simulink library "downlink_4c2t_foldingcfr_3firs_lib"  (Simulink 8.7)
settings: Solver=ode45  StartTime=0.0  StopTime=10.0  RelTol=1e-3
undefined symbols (not defined in the file or in its folder): AdvDSPBChannelOutDisplay, Anti, cfr_Params, dpoly, dspba_ChannelInVis, dspba_ChannelOutVis, dspba_internal_get_channel_ports, evalAionMaskParam, Folding, latency, primtype, REG, Symmetrical, value
undefined symbols (not defined in the file): cfr0_id, cfr_angle_cord_bits, cfr_angle_cord_fractional_bits, cfr_stages, cfr_xy_cord_bits, cfr_xy_cord_fractional_bits, clock_rate, DUC_LINEUP_param, REG_dut_id_addr, sample_rate
libraries: DSPBAPrim x74, CORDIC_lib x18, FoldingCFR_3FIRs_lib x16, DSPBAFilters x4, DSPBAModelBus x3, DSPBABase x3
(part 1 of 2)
settings Model: Creator=nsafari  LastModifiedBy=5g

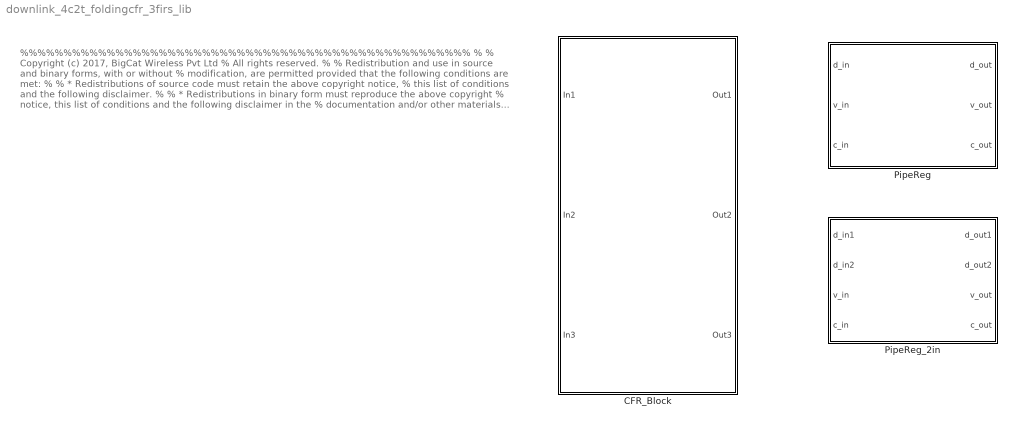
== system downlink_4c2t_foldingcfr_3firs_lib ==
  note: %%%%%%%%%%%%%%%%%%%%%%%%%%%%%%%%%%%%%%%%%%%%%%%%%%%%
      |  %
      |  % Copyright (c) 2017, BigCat Wireless Pvt Ltd
      |  % All rights reserved.
      |  %
      |  % Redistribution and use in source and binary forms, with or without
      |  % modification, are permitted provided that the following conditions are met:
      |  %
      |  %     * Redistributions of source code must retain the above copyright notice,
      |  %       this list of conditions and the following disclaimer.
      |  %
      |  %     * Redistributions in binary form must reproduce the above copyright
      |  %       notice, this list of conditions and the following disclaimer in the
      |  %       documentation and/or other materials provided with the distribution.
      |  %
      |  %     * Neither the name of the copyright holder nor the names of its contributors
      |  %       may be used to endorse or promote products derived from this software
      |  %       without specific prior written permission.
      |  %
      |  %
      |  %
      |  % THIS SOFTWARE IS PROVIDED BY THE COPYRIGHT HOLDERS AND CONTRIBUTORS "AS IS"
      |  % AND ANY EXPRESS OR IMPLIED WARRANTIES, INCLUDING, BUT NOT LIMITED TO, THE
      |  % IMPLIED WARRANTIES OF MERCHANTABILITY AND FITNESS FOR A PARTICULAR PURPOSE ARE
      |  % DISCLAIMED. IN NO EVENT SHALL THE COPYRIGHT HOLDER OR CONTRIBUTORS BE LIABLE
      |  % FOR ANY DIRECT, INDIRECT, INCIDENTAL, SPECIAL, EXEMPLARY, OR CONSEQUENTIAL
      |  % DAMAGES (INCLUDING, BUT NOT LIMITED TO, PROCUREMENT OF SUBSTITUTE GOODS OR
      |  % SERVICES; LOSS OF USE, DATA, OR PROFITS; OR BUSINESS INTERRUPTION) HOWEVER
      |  % CAUSED AND ON ANY THEORY OF LIABILITY, WHETHER IN CONTRACT, STRICT LIABILITY,
      |  % OR TORT (INCLUDING NEGLIGENCE OR OTHERWISE) ARISING IN ANY WAY OUT OF THE USE
      |  % OF THIS SOFTWARE, EVEN IF ADVISED OF THE POSSIBILITY OF SUCH DAMAGE.
      |  %
      |   %%%%%%%%%%%%%%%%%%%%%%%%%%%%%%%%%%%%%%%%%%%%%%%%%%%%%
  CFR_Block : Subsystem  AncestorBlock=CFR_library/CFR_Block  mask(Altera CFR Library Block){clk=clock_rate, sample_rate=sample_rate, Folding=Folding, block_id=cfr0_id, block_id_addr=REG_dut_id_addr, cfr_Params=cfr_Params, REG=REG}
      mask prompts: clk "System clock"; sample_rate "sample rate"; Folding "Folding Factor"; block_id "Unique ID of CFR"; block_id_addr "CFR ID address"; cfr_Params "CFR Configuration Structure"; REG "Register Map"
      mask help:
      | The block has the following parameters:
      |
      | "system clock" - the clock rate CFR module runs.
      |
      | "sample rate" - input signal sampling rate.
      |
      | "Folding Factor" - the number of folding for the module time-sharing;
      | It takes integer values between 1 and floor(system clock / sample rate).
      |
      | "Unique ID of CFR" is a unique numerical integer identifier for the CFR
      | block, this is used once the block is in a larger system to confirm the
      | correct block is being accessed.
      |
      | "CFR ID address" this is the relative address of the "Unique ID of CFR"
      | typically this is zero (at the CFR base address).
      |
      | "CFR Configuration Structure" - an array structure containing the
      | configuration of the CFR block. The length of this parameter specifies the
      | number of CFR core iterations instantiated.
      |
      | "Register Map" a structure containing the register map for CFR block.
      |
      | The settings of the above are exemplified in the setup script of the
      | altera_cfr example design.
      mask init:
      | %setup_cfr_block(iters, Iter_Params, REG, block_id, block_id_addr);
      mask Display:
      | color('w');
      | image(imread('dspba_prim.jpg'));
      | fprintf('FIR-based \n Peak Cancelling CFR \n \n Folding Factor: %d\n', Folding);
      | port_label('input',1,'valid');port_label('input',2,'channel');port_label('input',3,'xr');
      | port_label('output',1,'v');port_label('output',2,'c');port_label('output',3,'zr');
  PipeReg : Subsystem  mask{NPipe=2, Clock_Margin=DUC_LINEUP_param.ClockMargin}
      mask prompts: NPipe "Pipeline stages"; Clock_Margin "Clock Margin"
      mask Display:
      | d = strcat(num2str(NPipe), '\npipeline\nstages');
      | disp(d);
      | port_label('input',2,'v_in');
      | port_label('input',3,'c_in');
      | port_label('input',1,'d_in');
      | port_label('output',2,'v_out');
      | port_label('output',3,'c_out');
      | port_label('output',1,'d_out');
  PipeReg_2in : Subsystem  mask{NPipe=2, Clock_Margin=DUC_LINEUP_param.ClockMargin}
      mask prompts: NPipe "Pipeline stages"; Clock_Margin "Clock Margin"
      mask Display:
      | d = strcat(num2str(NPipe), '\npipeline\nstages');
      | disp(d);
      | port_label('input',3,'v_in');
      | port_label('input',4,'c_in');
      | port_label('input',1,'d_in1');
      | port_label('input',2,'d_in2');
      | port_label('output',3,'v_out');
      | port_label('output',4,'c_out');
      | port_label('output',1,'d_out1');
      | port_label('output',2,'d_out2');

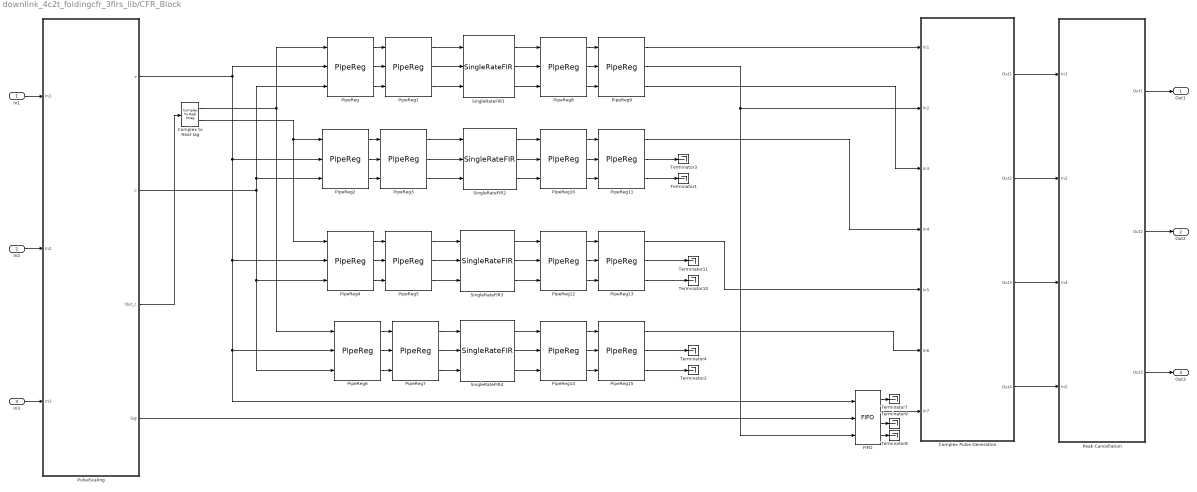
== system downlink_4c2t_foldingcfr_3firs_lib/CFR_Block ==
  In1 : Inport
  In2 : Inport  Port=2
  In3 : Inport  Port=3
  Complex Pulse Generation : Subsystem
  Complex to Real-Iag : ComplexToRealImag
  FIFO : DSPBAPrim/FIFO  primtype=fifo  nInputs=3  nOutputs=4  omode=Inherit via internal rule  otype=sfix(16)  scale=2^-15  rndmethod=Unbiased  factor=1  satmethod=Symmetric  shift_vec=[0 1 2 -1]  value=[16 8 16]  inPortNames=['w'; 'd'; 'r'; 'f']  outPortNames=['v'; 'q'; 't'; 'f']  dspbaimage=dspba_prim.jpg  text=fprintf('fifo');  style=Optimised  visibilities=263168  version=20130808  user_sclr=off
  Peak Cancellation : Subsystem
  PipeReg{,1..15} (16 alike) : FoldingCFR_3FIRs_lib/PipeReg  NPipe=2  Clock_Margin=DUC_LINEUP_param.ClockMargin
  PulseScaling : Subsystem
  SingleRateFIR1 : DSPBAFilters/SingleRateFIR  nInputRate=sample_rate  nchan=Folding  symmetry=Symmetrical  coef=fi(cfr_Params.firCOEF1,1,16,15)  addr=cfr_Params.BaseAddr + REG.FirTap1  rwmode=Read/Write  nband=Use All Taps  latency=3  exposebus=off  version=20090407
      settings: AttributesFormatString=%<latency>
  SingleRateFIR2 : DSPBAFilters/SingleRateFIR  nInputRate=sample_rate  nchan=Folding  symmetry=Anti-Symmetrical  coef=fi(cfr_Params.firCOEF2,1,16,15)  addr=cfr_Params.BaseAddr + REG.FirTap2  rwmode=Read/Write  nband=Use All Taps  latency=3  exposebus=off  version=20090407
  SingleRateFIR3 : DSPBAFilters/SingleRateFIR  nInputRate=sample_rate  nchan=Folding  symmetry=Symmetrical  coef=fi(cfr_Params.firCOEF3,1,16,15)  addr=cfr_Params.BaseAddr + REG.FirTap3  rwmode=Read/Write  nband=Use All Taps  latency=3  exposebus=off  version=20090407
  SingleRateFIR4 : DSPBAFilters/SingleRateFIR  nInputRate=sample_rate  nchan=Folding  symmetry=Anti-Symmetrical  coef=fi(cfr_Params.firCOEF4,1,16,15)  addr=cfr_Params.BaseAddr + REG.FirTap4  rwmode=Read/Write  nband=Use All Taps  latency=3  exposebus=off  version=20090407
  Terminator{1..4,7..11} (9 alike) : Terminator
  Out1 : Outport
  Out2 : Outport  Port=2
  Out3 : Outport  Port=3
  wires:
  In1/1 -> PulseScaling/1(In1)
  In2/1 -> PulseScaling/2(In2)
  In3/1 -> PulseScaling/3(In3)
  Peak Cancellation/1(Out1) -> Out1/1
  Peak Cancellation/2(Out2) -> Out2/1
  Peak Cancellation/3(Out3) -> Out3/1
  FIFO/1 -> Terminator7/1
  FIFO/4 -> Terminator8/1
  FIFO/3 -> Terminator9/1
  PulseScaling/3(Out_c) -> Complex to Real-Iag/1
  FIFO/2 -> Complex Pulse Generation/7(In7)
  Complex Pulse Generation/1(Out1) -> Peak Cancellation/1(In1)
  Complex Pulse Generation/3(Out3) -> Peak Cancellation/3(In4)
  Complex Pulse Generation/4(Out4) -> Peak Cancellation/4(In5)
  Complex Pulse Generation/2(Out2) -> Peak Cancellation/2(In2)
  Complex to Real-Iag/2 -> PipeReg4/1, PipeReg2/1
  Complex to Real-Iag/1 -> PipeReg6/1, PipeReg/1
  PulseScaling/2(c) -> PipeReg2/3, PipeReg/3, PipeReg6/3, PipeReg4/3
  PulseScaling/1(v) -> PipeReg/2, PipeReg4/2, PipeReg6/2, FIFO/1, PipeReg2/2
  PulseScaling/4(Sig) -> FIFO/2
  PipeReg9/3 -> Complex Pulse Generation/3(In3)
  PipeReg9/1 -> Complex Pulse Generation/1(In1)
  PipeReg9/2 -> FIFO/3, Complex Pulse Generation/2(In2)
  PipeReg11/1 -> Complex Pulse Generation/4(In4)
  PipeReg11/3 -> Terminator1/1
  PipeReg11/2 -> Terminator3/1
  PipeReg13/1 -> Complex Pulse Generation/5(In5)
  PipeReg13/3 -> Terminator10/1
  PipeReg13/2 -> Terminator11/1
  PipeReg15/1 -> Complex Pulse Generation/6(In6)
  PipeReg15/3 -> Terminator2/1
  PipeReg15/2 -> Terminator4/1
  PipeReg/3 -> PipeReg1/3
  PipeReg/1 -> PipeReg1/1
  PipeReg/2 -> PipeReg1/2
  PipeReg1/2 -> SingleRateFIR1/2
  PipeReg1/1 -> SingleRateFIR1/1
  PipeReg1/3 -> SingleRateFIR1/3
  PipeReg2/3 -> PipeReg3/3
  PipeReg2/1 -> PipeReg3/1
  PipeReg2/2 -> PipeReg3/2
  PipeReg3/1 -> SingleRateFIR2/1
  PipeReg3/2 -> SingleRateFIR2/2
  PipeReg3/3 -> SingleRateFIR2/3
  PipeReg4/3 -> PipeReg5/3
  PipeReg4/1 -> PipeReg5/1
  PipeReg4/2 -> PipeReg5/2
  PipeReg5/3 -> SingleRateFIR3/3
  PipeReg5/1 -> SingleRateFIR3/1
  PipeReg5/2 -> SingleRateFIR3/2
  PipeReg6/3 -> PipeReg7/3
  PipeReg6/1 -> PipeReg7/1
  PipeReg6/2 -> PipeReg7/2
  PipeReg7/1 -> SingleRateFIR4/1
  PipeReg7/2 -> SingleRateFIR4/2
  PipeReg7/3 -> SingleRateFIR4/3
  PipeReg8/3 -> PipeReg9/3
  PipeReg8/1 -> PipeReg9/1
  PipeReg8/2 -> PipeReg9/2
  SingleRateFIR1/1 -> PipeReg8/1
  SingleRateFIR1/3 -> PipeReg8/3
  SingleRateFIR1/2 -> PipeReg8/2
  PipeReg10/3 -> PipeReg11/3
  PipeReg10/1 -> PipeReg11/1
  PipeReg10/2 -> PipeReg11/2
  SingleRateFIR2/1 -> PipeReg10/1
  SingleRateFIR2/2 -> PipeReg10/2
  SingleRateFIR2/3 -> PipeReg10/3
  PipeReg12/3 -> PipeReg13/3
  PipeReg12/1 -> PipeReg13/1
  PipeReg12/2 -> PipeReg13/2
  SingleRateFIR3/2 -> PipeReg12/2
  SingleRateFIR3/1 -> PipeReg12/1
  SingleRateFIR3/3 -> PipeReg12/3
  PipeReg14/3 -> PipeReg15/3
  PipeReg14/1 -> PipeReg15/1
  PipeReg14/2 -> PipeReg15/2
  SingleRateFIR4/1 -> PipeReg14/1
  SingleRateFIR4/3 -> PipeReg14/3
  SingleRateFIR4/2 -> PipeReg14/2

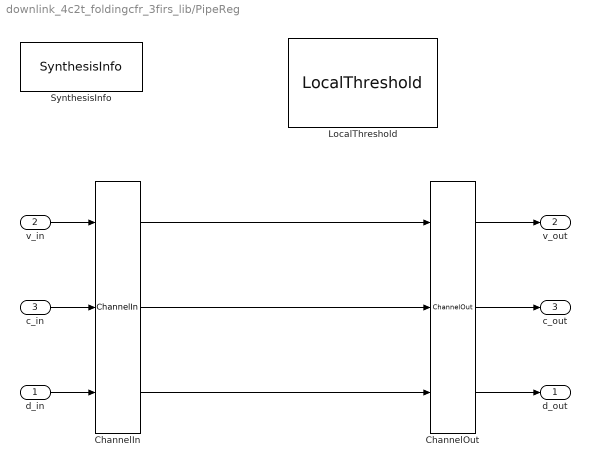
== system downlink_4c2t_foldingcfr_3firs_lib/PipeReg ==
  d_in : Inport
  v_in : Inport  Port=2
  c_in : Inport  Port=3
  ChannelIn : DSPBAPrim/ChannelIn  primtype=channelin  nInputs=dspba_internal_get_channel_ports(gcb)  nOutputs=dspba_internal_get_channel_ports(gcb)  omode=Inherit via internal rule  otype=sfix(16)  scale=2^-15  rndmethod=Unbiased  factor=1  satmethod=Symmetric  shift_vec=[0 1 2 -1]  value=1  inPortNames=['v'; 'c'; '0'; '1'; '2'; '3'; '4'; '5'; '6'; '7'; '8'; '9'; 'A'; 'B'; 'D'; 'E'; 'F'; 'G'; 'H'; 'I'; 'J'; 'K'; 'L'; 'M'; 'N'; 'O'; 'P'; 'Q'; 'R'; 'S'; 'T'; 'U'; 'W'; 'X'; 'Y'; 'Z']  outPortNames=['v'; 'c'; '0'; '1'; '2'; '3'; '4'; '5'; '6'; '7'; '8'; '9'; 'A'; 'B'; 'D'; 'E'; 'F'; 'G'; 'H'; 'I'; 'J'; 'K'; 'L'; 'M'; 'N'; 'O'; 'P'; 'Q'; 'R'; 'S'; 'T'; 'U'; 'W'; 'X'; 'Y'; 'Z']  dspbaimage=dspba_prim.jpg  text=fprintf('In');  style=Optimised  dataSignals=1  foldingEnabled=off  channels=1  sampleRate=200  packetBeginPresent=off  packetBeginEnabled=off  visibilities=dspba_ChannelInVis(gcb)  latencyCorrection=0  version=20141013
  ChannelOut : DSPBAPrim/ChannelOut  primtype=channelout  nInputs=dspba_internal_get_channel_ports(gcb)  nOutputs=dspba_internal_get_channel_ports(gcb)  omode=Inherit via internal rule  otype=sfix(16)  scale=2^-15  rndmethod=Unbiased  factor=1  satmethod=Symmetric  shift_vec=[0 1 2 -1]  value=1  inPortNames=['v'; 'c'; '0'; '1'; '2'; '3'; '4'; '5'; '6'; '7'; '8'; '9'; 'A'; 'B'; 'D'; 'E'; 'F'; 'G'; 'H'; 'I'; 'J'; 'K'; 'L'; 'M'; 'N'; 'O'; 'P'; 'Q'; 'R'; 'S'; 'T'; 'U'; 'W'; 'X'; 'Y'; 'Z']  outPortNames=['v'; 'c'; '0'; '1'; '2'; '3'; '4'; '5'; '6'; '7'; '8'; '9'; 'A'; 'B'; 'D'; 'E'; 'F'; 'G'; 'H'; 'I'; 'J'; 'K'; 'L'; 'M'; 'N'; 'O'; 'P'; 'Q'; 'R'; 'S'; 'T'; 'U'; 'W'; 'X'; 'Y'; 'Z']  dspbaimage=dspba_prim.jpg  text=fprintf('Out%s', AdvDSPBChannelOutDisplay(latency));  style=Optimised  dataSignals=1  foldingEnabled=off  channels=1  sampleRate=200  packetBeginPresent=off  packetBeginEnabled=off  visibilities=dspba_ChannelOutVis(gcb)  latency=2  latencyCorrection=0  version=20141013
  LocalThreshold : DSPBABase/LocalThreshold  margin=Clock_Margin  delayRegOrRAMThresholdBits=10000  MediumDualMemThresholdBits=-1  LargeDualMemThresholdBits=-1  hardMultiplierThresholdLuts=-1  version=0
  SynthesisInfo : DSPBAPrim/SynthesisInfo  primtype=synthinfo  nInputs=0  nOutputs=0  omode=Inherit via internal rule  otype=sfix(16)  scale=2^-15  rndmethod=Truncate  factor=1  satmethod=Symmetric  shift_vec=[0 1 2 -1]  value=99  inPortNames=[' '; ' ';]  outPortNames=[' ']  dspbaimage=dspba_prim.jpg  text=fprintf('Style=%s', style);  style=Scheduled  visibilities=32768  constraintInUse=on  constraintRelation==  constraintLimit=NPipe  bitAccurate=off  version=20090407
  d_out : Outport
  v_out : Outport  Port=2
  c_out : Outport  Port=3
  wires:
  ChannelOut/2 -> c_out/1
  ChannelOut/1 -> v_out/1
  ChannelOut/3 -> d_out/1
  c_in/1 -> ChannelIn/2
  v_in/1 -> ChannelIn/1
  ChannelIn/2 -> ChannelOut/2
  d_in/1 -> ChannelIn/3
  ChannelIn/1 -> ChannelOut/1
  ChannelIn/3 -> ChannelOut/3

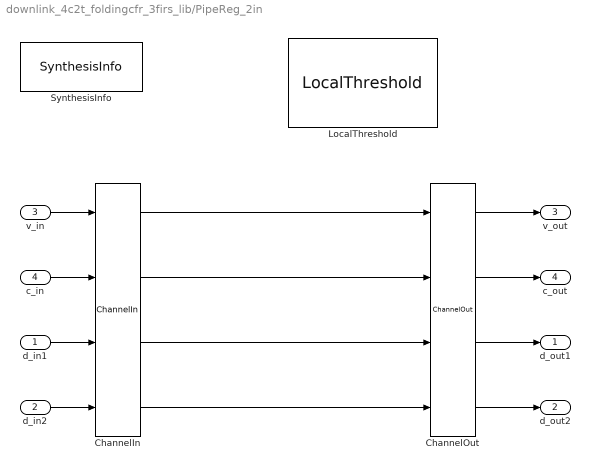
== system downlink_4c2t_foldingcfr_3firs_lib/PipeReg_2in ==
  d_in1 : Inport
  d_in2 : Inport  Port=2
  v_in : Inport  Port=3
  c_in : Inport  Port=4
  ChannelIn : DSPBAPrim/ChannelIn  primtype=channelin  nInputs=dspba_internal_get_channel_ports(gcb)  nOutputs=dspba_internal_get_channel_ports(gcb)  omode=Inherit via internal rule  otype=sfix(16)  scale=2^-15  rndmethod=Unbiased  factor=1  satmethod=Symmetric  shift_vec=[0 1 2 -1]  value=2  inPortNames=['v'; 'c'; '0'; '1'; '2'; '3'; '4'; '5'; '6'; '7'; '8'; '9'; 'A'; 'B'; 'D'; 'E'; 'F'; 'G'; 'H'; 'I'; 'J'; 'K'; 'L'; 'M'; 'N'; 'O'; 'P'; 'Q'; 'R'; 'S'; 'T'; 'U'; 'W'; 'X'; 'Y'; 'Z']  outPortNames=['v'; 'c'; '0'; '1'; '2'; '3'; '4'; '5'; '6'; '7'; '8'; '9'; 'A'; 'B'; 'D'; 'E'; 'F'; 'G'; 'H'; 'I'; 'J'; 'K'; 'L'; 'M'; 'N'; 'O'; 'P'; 'Q'; 'R'; 'S'; 'T'; 'U'; 'W'; 'X'; 'Y'; 'Z']  dspbaimage=dspba_prim.jpg  text=fprintf('In');  style=Optimised  dataSignals=2  foldingEnabled=off  channels=1  sampleRate=200  packetBeginPresent=off  packetBeginEnabled=off  visibilities=dspba_ChannelInVis(gcb)  latencyCorrection=0  version=20141013
  ChannelOut : DSPBAPrim/ChannelOut  primtype=channelout  nInputs=dspba_internal_get_channel_ports(gcb)  nOutputs=dspba_internal_get_channel_ports(gcb)  omode=Inherit via internal rule  otype=sfix(16)  scale=2^-15  rndmethod=Unbiased  factor=1  satmethod=Symmetric  shift_vec=[0 1 2 -1]  value=2  inPortNames=['v'; 'c'; '0'; '1'; '2'; '3'; '4'; '5'; '6'; '7'; '8'; '9'; 'A'; 'B'; 'D'; 'E'; 'F'; 'G'; 'H'; 'I'; 'J'; 'K'; 'L'; 'M'; 'N'; 'O'; 'P'; 'Q'; 'R'; 'S'; 'T'; 'U'; 'W'; 'X'; 'Y'; 'Z']  outPortNames=['v'; 'c'; '0'; '1'; '2'; '3'; '4'; '5'; '6'; '7'; '8'; '9'; 'A'; 'B'; 'D'; 'E'; 'F'; 'G'; 'H'; 'I'; 'J'; 'K'; 'L'; 'M'; 'N'; 'O'; 'P'; 'Q'; 'R'; 'S'; 'T'; 'U'; 'W'; 'X'; 'Y'; 'Z']  dspbaimage=dspba_prim.jpg  text=fprintf('Out%s', AdvDSPBChannelOutDisplay(latency));  style=Optimised  dataSignals=2  foldingEnabled=off  channels=1  sampleRate=200  packetBeginPresent=off  packetBeginEnabled=off  visibilities=dspba_ChannelOutVis(gcb)  latency=2  latencyCorrection=0  version=20141013
  LocalThreshold : DSPBABase/LocalThreshold  margin=Clock_Margin  delayRegOrRAMThresholdBits=10000  MediumDualMemThresholdBits=-1  LargeDualMemThresholdBits=-1  hardMultiplierThresholdLuts=-1  version=0
  SynthesisInfo : DSPBAPrim/SynthesisInfo  primtype=synthinfo  nInputs=0  nOutputs=0  omode=Inherit via internal rule  otype=sfix(16)  scale=2^-15  rndmethod=Truncate  factor=1  satmethod=Symmetric  shift_vec=[0 1 2 -1]  value=99  inPortNames=[' '; ' ';]  outPortNames=[' ']  dspbaimage=dspba_prim.jpg  text=fprintf('Style=%s', style);  style=Scheduled  visibilities=32768  constraintInUse=on  constraintRelation==  constraintLimit=NPipe  bitAccurate=off  version=20090407
  "d_out1 " : Outport
  d_out2 : Outport  Port=2
  v_out : Outport  Port=3
  c_out : Outport  Port=4
  wires:
  ChannelIn/3 -> ChannelOut/3
  ChannelIn/1 -> ChannelOut/1
  d_in1/1 -> ChannelIn/3
  ChannelIn/2 -> ChannelOut/2
  v_in/1 -> ChannelIn/1
  c_in/1 -> ChannelIn/2
  ChannelOut/3 -> "d_out1 "/1
  ChannelOut/1 -> v_out/1
  ChannelOut/2 -> c_out/1
  d_in2/1 -> ChannelIn/4
  ChannelIn/4 -> ChannelOut/4
  ChannelOut/4 -> d_out2/1

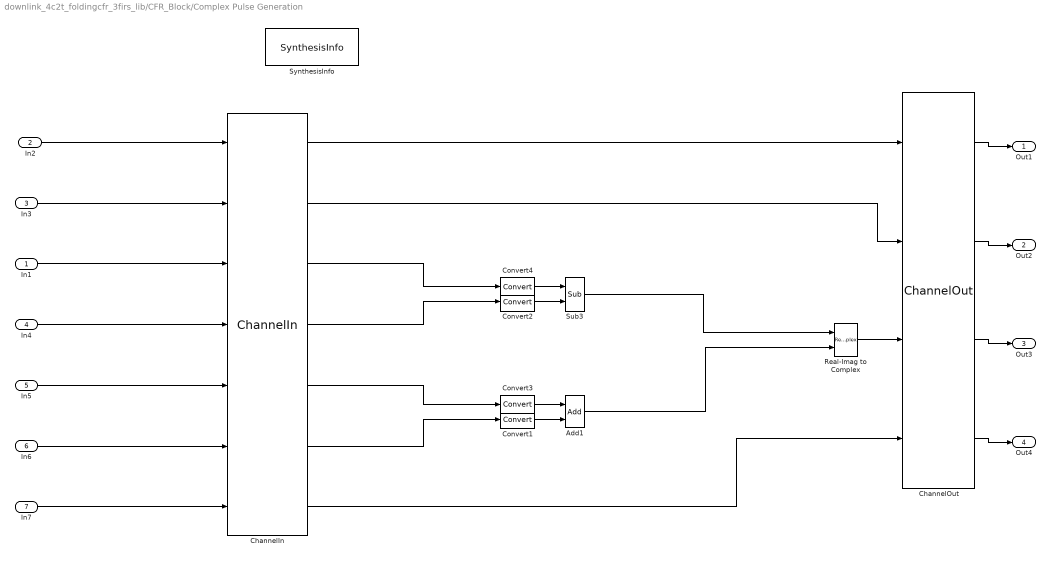
== system downlink_4c2t_foldingcfr_3firs_lib/CFR_Block/Complex Pulse Generation ==
  In1 : Inport
  In2 : Inport  Port=2
  In3 : Inport  Port=3
  In4 : Inport  Port=4
  In5 : Inport  Port=5
  In6 : Inport  Port=6
  In7 : Inport  Port=7
  Add1 : DSPBAPrim/Add  primtype=add  nInputs=evalAionMaskParam(gcb,'value',1)  nOutputs=1  omode=Inherit via internal rule with word growth  otype=sfix(16)  scale=2^-15  rndmethod=Unbiased  factor=1  satmethod=Symmetric  shift_vec=[0 1 2 -1]  value=2  inPortNames=[' '; ' ';]  outPortNames=[' ']  dspbaimage=dspba_prim.jpg  text=fprintf('+');  style=Optimised  visibilities=1032+2^17+2^18+2^19  genFPC=off  floatRounding=correct  advOptions=[]  version=20130821
  ChannelIn : DSPBAPrim/ChannelIn  primtype=channelin  nInputs=dspba_internal_get_channel_ports(gcb)  nOutputs=dspba_internal_get_channel_ports(gcb)  omode=Inherit via internal rule  otype=sfix(16)  scale=2^-15  rndmethod=Unbiased  factor=1  satmethod=Symmetric  shift_vec=[0 1 2 -1]  value=5  inPortNames=['v'; 'c'; '0'; '1'; '2'; '3'; '4'; '5'; '6'; '7'; '8'; '9'; 'A'; 'B'; 'D'; 'E'; 'F'; 'G'; 'H'; 'I'; 'J'; 'K'; 'L'; 'M'; 'N'; 'O'; 'P'; 'Q'; 'R'; 'S'; 'T'; 'U'; 'W'; 'X'; 'Y'; 'Z']  outPortNames=['v'; 'c'; '0'; '1'; '2'; '3'; '4'; '5'; '6'; '7'; '8'; '9'; 'A'; 'B'; 'D'; 'E'; 'F'; 'G'; 'H'; 'I'; 'J'; 'K'; 'L'; 'M'; 'N'; 'O'; 'P'; 'Q'; 'R'; 'S'; 'T'; 'U'; 'W'; 'X'; 'Y'; 'Z']  dspbaimage=dspba_prim.jpg  text=fprintf('In');  style=Optimised  dataSignals=5  foldingEnabled=off  channels=1  sampleRate=200  packetBeginPresent=off  packetBeginEnabled=off  visibilities=dspba_ChannelInVis(gcb)  latencyCorrection=0  version=20141013
  ChannelOut : DSPBAPrim/ChannelOut  primtype=channelout  nInputs=dspba_internal_get_channel_ports(gcb)  nOutputs=dspba_internal_get_channel_ports(gcb)  omode=Inherit via internal rule  otype=sfix(16)  scale=2^-15  rndmethod=Unbiased  factor=1  satmethod=Symmetric  shift_vec=[0 1 2 -1]  value=2  inPortNames=['v'; 'c'; '0'; '1'; '2'; '3'; '4'; '5'; '6'; '7'; '8'; '9'; 'A'; 'B'; 'D'; 'E'; 'F'; 'G'; 'H'; 'I'; 'J'; 'K'; 'L'; 'M'; 'N'; 'O'; 'P'; 'Q'; 'R'; 'S'; 'T'; 'U'; 'W'; 'X'; 'Y'; 'Z']  outPortNames=['v'; 'c'; '0'; '1'; '2'; '3'; '4'; '5'; '6'; '7'; '8'; '9'; 'A'; 'B'; 'D'; 'E'; 'F'; 'G'; 'H'; 'I'; 'J'; 'K'; 'L'; 'M'; 'N'; 'O'; 'P'; 'Q'; 'R'; 'S'; 'T'; 'U'; 'W'; 'X'; 'Y'; 'Z']  dspbaimage=dspba_prim.jpg  text=fprintf('Out%s', AdvDSPBChannelOutDisplay(latency));  style=Optimised  dataSignals=2  foldingEnabled=off  channels=1  sampleRate=200  packetBeginPresent=off  packetBeginEnabled=off  visibilities=dspba_ChannelOutVis(gcb)  latency=6  latencyCorrection=0  version=20141013
  Convert{1..4} (4 alike) : DSPBAPrim/Convert  primtype=convert  nInputs=1  nOutputs=1  omode=Specify via dialog  otype=sfix(16)  scale=2^-15  rndmethod=Unbiased  factor=1  satmethod=None  shift_vec=[0 1 2 -1]  value=round([0:255]/17)  inPortNames=[' '; ' ';]  outPortNames=[' '; 'c']  dspbaimage=dspba_prim.jpg  text=fprintf('convert');  style=Optimised  visibilities=8+64+256+2^17  clipdetect=off  floatPrecision=float32_m23  advOptions=[]  version=20130211
  Real-Imag to Complex : RealImagToComplex
  Sub3 : DSPBAPrim/Sub  primtype=sub  nInputs=2  nOutputs=1  omode=Inherit via internal rule with word growth  otype=sfix(16)  scale=2^-15  rndmethod=Unbiased  factor=1  satmethod=Symmetric  shift_vec=[0 1 2 -1]  value=0  inPortNames=['+'; '-';]  outPortNames=[' ']  dspbaimage=dspba_prim.jpg  text=fprintf('-');  style=Optimised  visibilities=8  floatRounding=correct  advOptions=[]  version=20130115
  SynthesisInfo : DSPBAPrim/SynthesisInfo  primtype=synthinfo  nInputs=0  nOutputs=0  omode=Inherit via internal rule  otype=sfix(16)  scale=2^-15  rndmethod=Truncate  factor=1  satmethod=Symmetric  shift_vec=[0 1 2 -1]  value=99  inPortNames=[' '; ' ';]  outPortNames=[' ']  dspbaimage=dspba_prim.jpg  text=fprintf('Style=%s', style);  style=Scheduled  visibilities=32768  constraintInUse=on  constraintRelation=>  constraintLimit=20  bitAccurate=off  version=20090407
  Out1 : Outport
  Out2 : Outport  Port=2
  Out3 : Outport  Port=3
  Out4 : Outport  Port=4
  wires:
  In1/1 -> ChannelIn/3
  ChannelIn/4 -> Convert2/1
  In4/1 -> ChannelIn/4
  ChannelIn/3 -> Convert4/1
  ChannelIn/6 -> Convert1/1
  In3/1 -> ChannelIn/2
  ChannelIn/1 -> ChannelOut/1
  ChannelIn/2 -> ChannelOut/2
  In7/1 -> ChannelIn/7
  ChannelIn/5 -> Convert3/1
  In5/1 -> ChannelIn/5
  In6/1 -> ChannelIn/6
  In2/1 -> ChannelIn/1
  ChannelIn/7 -> ChannelOut/4
  Sub3/1 -> Real-Imag to Complex/1
  ChannelOut/1 -> Out1/1
  ChannelOut/4 -> Out4/1
  ChannelOut/3 -> Out3/1
  Real-Imag to Complex/1 -> ChannelOut/3
  Add1/1 -> Real-Imag to Complex/2
  Convert1/1 -> Add1/2
  Convert3/1 -> Add1/1
  Convert2/1 -> Sub3/2
  Convert4/1 -> Sub3/1
  ChannelOut/2 -> Out2/1

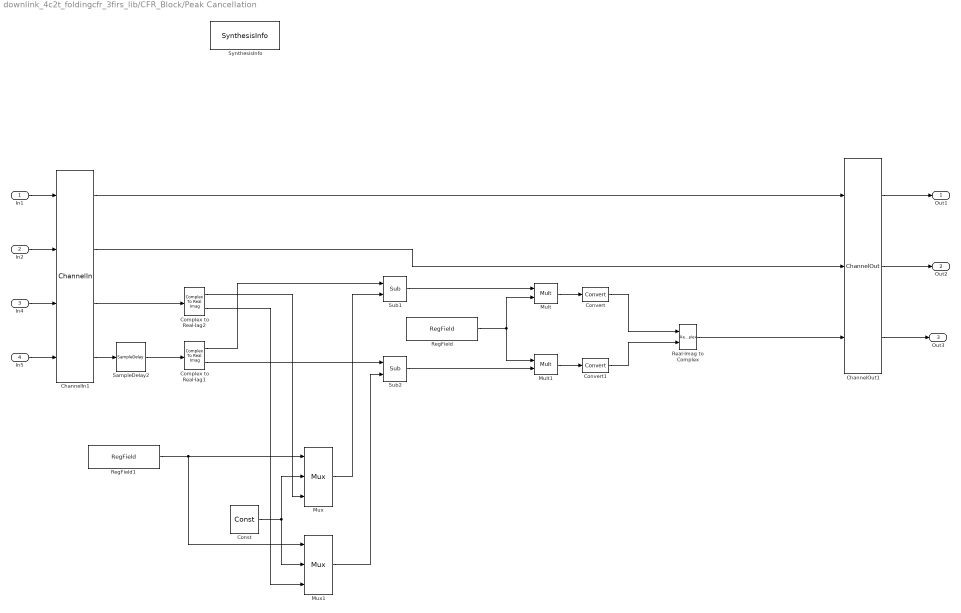
== system downlink_4c2t_foldingcfr_3firs_lib/CFR_Block/Peak Cancellation ==
  In1 : Inport
  In2 : Inport  Port=2
  In4 : Inport  Port=3
  In5 : Inport  Port=4
  ChannelIn1 : DSPBAPrim/ChannelIn  primtype=channelin  nInputs=dspba_internal_get_channel_ports(gcb)  nOutputs=dspba_internal_get_channel_ports(gcb)  omode=Inherit via internal rule  otype=sfix(16)  scale=2^-15  rndmethod=Unbiased  factor=1  satmethod=Symmetric  shift_vec=[0 1 2 -1]  value=2  inPortNames=['v'; 'c'; '0'; '1'; '2'; '3'; '4'; '5'; '6'; '7'; '8'; '9'; 'A'; 'B'; 'D'; 'E'; 'F'; 'G'; 'H'; 'I'; 'J'; 'K'; 'L'; 'M'; 'N'; 'O'; 'P'; 'Q'; 'R'; 'S'; 'T'; 'U'; 'W'; 'X'; 'Y'; 'Z']  outPortNames=['v'; 'c'; '0'; '1'; '2'; '3'; '4'; '5'; '6'; '7'; '8'; '9'; 'A'; 'B'; 'D'; 'E'; 'F'; 'G'; 'H'; 'I'; 'J'; 'K'; 'L'; 'M'; 'N'; 'O'; 'P'; 'Q'; 'R'; 'S'; 'T'; 'U'; 'W'; 'X'; 'Y'; 'Z']  dspbaimage=dspba_prim.jpg  text=fprintf('In');  style=Optimised  dataSignals=2  foldingEnabled=off  channels=1  sampleRate=200  packetBeginPresent=off  packetBeginEnabled=off  visibilities=dspba_ChannelInVis(gcb)  latencyCorrection=0  version=20141013
  ChannelOut1 : DSPBAPrim/ChannelOut  primtype=channelout  nInputs=dspba_internal_get_channel_ports(gcb)  nOutputs=dspba_internal_get_channel_ports(gcb)  omode=Inherit via internal rule  otype=sfix(16)  scale=2^-15  rndmethod=Unbiased  factor=1  satmethod=Symmetric  shift_vec=[0 1 2 -1]  value=1  inPortNames=['v'; 'c'; '0'; '1'; '2'; '3'; '4'; '5'; '6'; '7'; '8'; '9'; 'A'; 'B'; 'D'; 'E'; 'F'; 'G'; 'H'; 'I'; 'J'; 'K'; 'L'; 'M'; 'N'; 'O'; 'P'; 'Q'; 'R'; 'S'; 'T'; 'U'; 'W'; 'X'; 'Y'; 'Z']  outPortNames=['v'; 'c'; '0'; '1'; '2'; '3'; '4'; '5'; '6'; '7'; '8'; '9'; 'A'; 'B'; 'D'; 'E'; 'F'; 'G'; 'H'; 'I'; 'J'; 'K'; 'L'; 'M'; 'N'; 'O'; 'P'; 'Q'; 'R'; 'S'; 'T'; 'U'; 'W'; 'X'; 'Y'; 'Z']  dspbaimage=dspba_prim.jpg  text=fprintf('Out%s', AdvDSPBChannelOutDisplay(latency));  style=Optimised  dataSignals=1  foldingEnabled=off  channels=1  sampleRate=200  packetBeginPresent=off  packetBeginEnabled=off  visibilities=dspba_ChannelOutVis(gcb)  latency=12  latencyCorrection=0  version=20141013
  Complex to Real-Iag1 : ComplexToRealImag
  Complex to Real-Iag2 : ComplexToRealImag
  Const : DSPBAPrim/Const  primtype=const  nInputs=0  nOutputs=1  omode=Inherit via internal rule  otype=sfix(16)  scale=2^-15  rndmethod=Unbiased  factor=1  satmethod=Symmetric  shift_vec=[0 1 2 -1]  value=0  inPortNames=['+'; '+';]  outPortNames=[' ']  dspbaimage=dspba_prim.jpg  text=fprintf('%s', num2str(value));  style=Optimised  visibilities=8 + 1024  floatPrecision=float32_m23  version=20120820
  Convert : DSPBAPrim/Convert  primtype=convert  nInputs=1  nOutputs=1  omode=Specify via dialog  otype=sfix(16)  scale=2^-15  rndmethod=Unbiased  factor=1  satmethod=None  shift_vec=[0 1 2 -1]  value=round([0:255]/17)  inPortNames=[' '; ' ';]  outPortNames=[' '; 'c']  dspbaimage=dspba_prim.jpg  text=fprintf('convert');  style=Optimised  visibilities=8+64+256+2^17  clipdetect=off  floatPrecision=float32_m23  advOptions=[]  version=20130211
  Convert1 : DSPBAPrim/Convert  primtype=convert  nInputs=1  nOutputs=1  omode=Specify via dialog  otype=sfix(16)  scale=2^-15  rndmethod=Unbiased  factor=1  satmethod=None  shift_vec=[0 1 2 -1]  value=round([0:255]/17)  inPortNames=[' '; ' ';]  outPortNames=[' '; 'c']  dspbaimage=dspba_prim.jpg  text=fprintf('convert');  style=Optimised  visibilities=8+64+256+2^17  clipdetect=off  floatPrecision=float32_m23  advOptions=[]  version=20130211
  Mult : DSPBAPrim/Mult  primtype=mult  nInputs=2  nOutputs=1  omode=Inherit via internal rule  otype=sfix(16)  scale=2^-15  rndmethod=Unbiased  factor=1  satmethod=Symmetric  shift_vec=[0 1 2 -1]  value=0  inPortNames=[' '; ' ';]  outPortNames=[' ']  dspbaimage=dspba_prim.jpg  text=fprintf('X');  style=Optimised  visibilities=8+2^18+2^19  floatPrecision=float32_m23  floatRounding=correct  advOptions=[]  version=20130115
  Mult1 : DSPBAPrim/Mult  primtype=mult  nInputs=2  nOutputs=1  omode=Inherit via internal rule  otype=sfix(16)  scale=2^-15  rndmethod=Unbiased  factor=1  satmethod=Symmetric  shift_vec=[0 1 2 -1]  value=0  inPortNames=[' '; ' ';]  outPortNames=[' ']  dspbaimage=dspba_prim.jpg  text=fprintf('X');  style=Optimised  visibilities=8+2^18+2^19  floatPrecision=float32_m23  floatRounding=correct  advOptions=[]  version=20130115
  Mux : DSPBAPrim/Mux  primtype=mux  nInputs=evalAionMaskParam(gcb,'value',1)+1  nOutputs=1  omode=Inherit via internal rule  otype=sfix(16)  scale=2^-15  rndmethod=Unbiased  factor=1  satmethod=Symmetric  shift_vec=[0 1 2 -1]  value=2  inPortNames=['s '; 'd0'; 'd1'; 'd2'; 'd3'; 'd4'; 'd5'; 'd6'; 'd7'; 'd8'; 'd9';]  outPortNames=[' ']  dspbaimage=dspba_prim.jpg  text=fprintf('%s', primtype);  style=Optimised  visibilities=1032  version=20131025
  Mux1 : DSPBAPrim/Mux  primtype=mux  nInputs=evalAionMaskParam(gcb,'value',1)+1  nOutputs=1  omode=Inherit via internal rule  otype=sfix(16)  scale=2^-15  rndmethod=Unbiased  factor=1  satmethod=Symmetric  shift_vec=[0 1 2 -1]  value=2  inPortNames=['s '; 'd0'; 'd1'; 'd2'; 'd3'; 'd4'; 'd5'; 'd6'; 'd7'; 'd8'; 'd9';]  outPortNames=[' ']  dspbaimage=dspba_prim.jpg  text=fprintf('%s', primtype);  style=Optimised  visibilities=1032  version=20131025
  Real-Imag to Complex : RealImagToComplex
  RegField : DSPBAModelBus/RegField  reg_name=cfr_Params.BaseAddr + REG.Scaling  reg_rwmode=Read/Write  reg_msb=15  reg_lsb=0  reg_mode=Specify via dialog  reg_type=ufix(16)  reg_scale=2^-12  reg_init=cfr_Params.Scaling  reg_desc=Scaling value  reg_modal=off  reg_desc0=0  reg_desc1=0  reg_desc2=0  reg_desc3=0  reg_desc4=0  reg_desc5=0  reg_desc6=0  reg_desc7=0  SampleTime=1  version=20090407
  RegField1 : DSPBAModelBus/RegField  reg_name=cfr_Params.BaseAddr + REG.Enable  reg_rwmode=Read/Write  reg_msb=0  reg_lsb=0  reg_mode=Specify via dialog  reg_type=ufix(1)  reg_scale=2^0  reg_init=cfr_Params.Enable  reg_desc=Enable CFR  reg_modal=off  reg_desc0=0  reg_desc1=0  reg_desc2=0  reg_desc3=0  reg_desc4=0  reg_desc5=0  reg_desc6=0  reg_desc7=0  SampleTime=1  version=20090407
  SampleDelay2 : DSPBAPrim/SampleDelay  primtype=sampdelay  nInputs=1  nOutputs=1  omode=Inherit via internal rule  otype=sfix(16)  scale=2^-15  rndmethod=Unbiased  factor=1  satmethod=Symmetric  shift_vec=[0 1 2 -1]  value=floor(length(cfr_Params.firCOEF1)/2)*Folding  inPortNames=[' '; ' ';]  outPortNames=[' ']  dspbaimage=dspba_prim.jpg  text=dpoly(1, eye(1,value+1), 'z')  style=Optimised  visibilities=8 + 1024 + 2^17 + 2^18  flexible=off  slackgroup=0  augmented=0  version=20090407  advOptions=[]
  Sub1 : DSPBAPrim/Sub  primtype=sub  nInputs=2  nOutputs=1  omode=Inherit via internal rule with word growth  otype=sfix(16)  scale=2^-15  rndmethod=Unbiased  factor=1  satmethod=Symmetric  shift_vec=[0 1 2 -1]  value=0  inPortNames=['+'; '-';]  outPortNames=[' ']  dspbaimage=dspba_prim.jpg  text=fprintf('-');  style=Optimised  visibilities=8  floatRounding=correct  advOptions=[]  version=20130115
  Sub2 : DSPBAPrim/Sub  primtype=sub  nInputs=2  nOutputs=1  omode=Inherit via internal rule with word growth  otype=sfix(16)  scale=2^-15  rndmethod=Unbiased  factor=1  satmethod=Symmetric  shift_vec=[0 1 2 -1]  value=0  inPortNames=['+'; '-';]  outPortNames=[' ']  dspbaimage=dspba_prim.jpg  text=fprintf('-');  style=Optimised  visibilities=8  floatRounding=correct  advOptions=[]  version=20130115
  SynthesisInfo : DSPBAPrim/SynthesisInfo  primtype=synthinfo  nInputs=0  nOutputs=0  omode=Inherit via internal rule  otype=sfix(16)  scale=2^-15  rndmethod=Truncate  factor=1  satmethod=Symmetric  shift_vec=[0 1 2 -1]  value=99  inPortNames=[' '; ' ';]  outPortNames=[' ']  dspbaimage=dspba_prim.jpg  text=fprintf('Style=%s', style);  style=Scheduled  visibilities=32768  constraintInUse=on  constraintRelation=>  constraintLimit=20  bitAccurate=off  version=20090407
  Out1 : Outport
  Out2 : Outport  Port=2
  Out3 : Outport  Port=3
  wires:
  ChannelIn1/3 -> Complex to Real-Iag2/1
  ChannelIn1/4 -> SampleDelay2/1
  Real-Imag to Complex/1 -> ChannelOut1/3
  ChannelIn1/1 -> ChannelOut1/1
  ChannelIn1/2 -> ChannelOut1/2
  In1/1 -> ChannelIn1/1
  In4/1 -> ChannelIn1/3
  In2/1 -> ChannelIn1/2
  In5/1 -> ChannelIn1/4
  ChannelOut1/1 -> Out1/1
  ChannelOut1/2 -> Out2/1
  ChannelOut1/3 -> Out3/1
  SampleDelay2/1 -> Complex to Real-Iag1/1
  RegField/1 -> Mult1/1, Mult/2
  Mult/1 -> Convert/1
  Mult1/1 -> Convert1/1
  Sub1/1 -> Mult/1
  Sub2/1 -> Mult1/2
  Convert/1 -> Real-Imag to Complex/1
  Convert1/1 -> Real-Imag to Complex/2
  RegField1/1 -> Mux/1, Mux1/1
  Complex to Real-Iag2/1 -> Mux/3
  Complex to Real-Iag2/2 -> Mux1/3
  Mux/1 -> Sub1/2
  Mux1/1 -> Sub2/2
  Const/1 -> Mux1/2, Mux/2
  Complex to Real-Iag1/1 -> Sub1/1
  Complex to Real-Iag1/2 -> Sub2/1

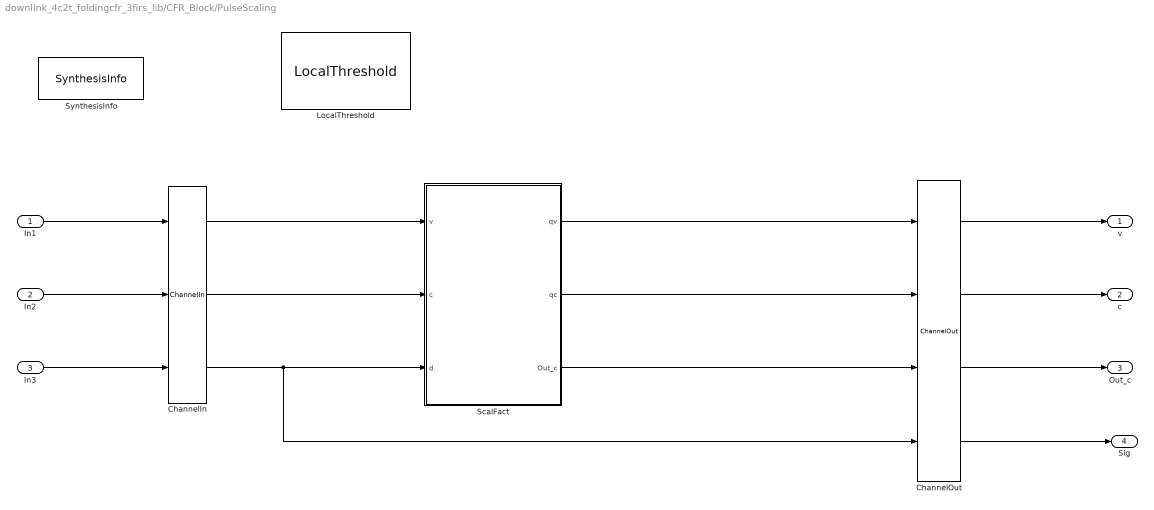
== system downlink_4c2t_foldingcfr_3firs_lib/CFR_Block/PulseScaling ==
  In1 : Inport
  In2 : Inport  Port=2
  In3 : Inport  Port=3
  ChannelIn : DSPBAPrim/ChannelIn  primtype=channelin  nInputs=dspba_internal_get_channel_ports(gcb)  nOutputs=dspba_internal_get_channel_ports(gcb)  omode=Inherit via internal rule  otype=sfix(16)  scale=2^-15  rndmethod=Unbiased  factor=1  satmethod=Symmetric  shift_vec=[0 1 2 -1]  value=1  inPortNames=['v'; 'c'; '0'; '1'; '2'; '3'; '4'; '5'; '6'; '7'; '8'; '9'; 'A'; 'B'; 'D'; 'E'; 'F'; 'G'; 'H'; 'I'; 'J'; 'K'; 'L'; 'M'; 'N'; 'O'; 'P'; 'Q'; 'R'; 'S'; 'T'; 'U'; 'W'; 'X'; 'Y'; 'Z']  outPortNames=['v'; 'c'; '0'; '1'; '2'; '3'; '4'; '5'; '6'; '7'; '8'; '9'; 'A'; 'B'; 'D'; 'E'; 'F'; 'G'; 'H'; 'I'; 'J'; 'K'; 'L'; 'M'; 'N'; 'O'; 'P'; 'Q'; 'R'; 'S'; 'T'; 'U'; 'W'; 'X'; 'Y'; 'Z']  dspbaimage=dspba_prim.jpg  text=fprintf('In');  style=Optimised  dataSignals=1  foldingEnabled=off  channels=1  sampleRate=200  packetBeginPresent=off  packetBeginEnabled=off  visibilities=dspba_ChannelInVis(gcb)  latencyCorrection=0  version=20141013
  ChannelOut : DSPBAPrim/ChannelOut  primtype=channelout  nInputs=dspba_internal_get_channel_ports(gcb)  nOutputs=dspba_internal_get_channel_ports(gcb)  omode=Inherit via internal rule  otype=sfix(16)  scale=2^-15  rndmethod=Unbiased  factor=1  satmethod=Symmetric  shift_vec=[0 1 2 -1]  value=2  inPortNames=['v'; 'c'; '0'; '1'; '2'; '3'; '4'; '5'; '6'; '7'; '8'; '9'; 'A'; 'B'; 'D'; 'E'; 'F'; 'G'; 'H'; 'I'; 'J'; 'K'; 'L'; 'M'; 'N'; 'O'; 'P'; 'Q'; 'R'; 'S'; 'T'; 'U'; 'W'; 'X'; 'Y'; 'Z']  outPortNames=['v'; 'c'; '0'; '1'; '2'; '3'; '4'; '5'; '6'; '7'; '8'; '9'; 'A'; 'B'; 'D'; 'E'; 'F'; 'G'; 'H'; 'I'; 'J'; 'K'; 'L'; 'M'; 'N'; 'O'; 'P'; 'Q'; 'R'; 'S'; 'T'; 'U'; 'W'; 'X'; 'Y'; 'Z']  dspbaimage=dspba_prim.jpg  text=fprintf('Out%s', AdvDSPBChannelOutDisplay(latency));  style=Optimised  dataSignals=2  foldingEnabled=off  channels=1  sampleRate=200  packetBeginPresent=off  packetBeginEnabled=off  visibilities=dspba_ChannelOutVis(gcb)  latency=82  latencyCorrection=0  version=20141013
  LocalThreshold : DSPBABase/LocalThreshold  margin=DUC_LINEUP_param.ClockMargin_CFR  delayRegOrRAMThresholdBits=-1  MediumDualMemThresholdBits=-1  LargeDualMemThresholdBits=-1  hardMultiplierThresholdLuts=-1  version=0
  ScalFact : Subsystem  mask{ClipVal=cfr_Params.ClipVal}
      mask prompts: ClipVal "cLipping Value"
  SynthesisInfo : DSPBAPrim/SynthesisInfo  primtype=synthinfo  nInputs=0  nOutputs=0  omode=Inherit via internal rule  otype=sfix(16)  scale=2^-15  rndmethod=Truncate  factor=1  satmethod=Symmetric  shift_vec=[0 1 2 -1]  value=99  inPortNames=[' '; ' ';]  outPortNames=[' ']  dspbaimage=dspba_prim.jpg  text=fprintf('Style=%s', style);  style=Scheduled  visibilities=32768  constraintInUse=on  constraintRelation=>  constraintLimit=100  bitAccurate=off  version=20090407
  v : Outport
  c : Outport  Port=2
  Out_c : Outport  Port=3
  Sig : Outport  Port=4
  wires:
  In1/1 -> ChannelIn/1
  In2/1 -> ChannelIn/2
  ScalFact/1(qv) -> ChannelOut/1
  ScalFact/2(qc) -> ChannelOut/2
  ScalFact/3(Out_c) -> ChannelOut/3
  In3/1 -> ChannelIn/3
  ChannelIn/1 -> ScalFact/1(v)
  ChannelIn/2 -> ScalFact/2(c)
  ChannelIn/3 -> ChannelOut/4, ScalFact/3(d)
  ChannelOut/1 -> v/1
  ChannelOut/2 -> c/1
  ChannelOut/3 -> Out_c/1
  ChannelOut/4 -> Sig/1

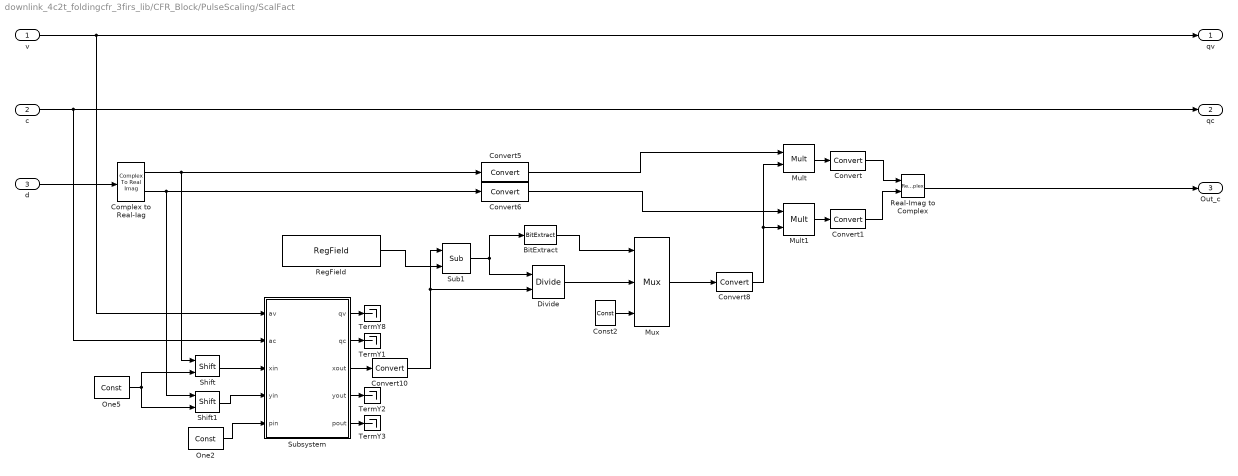
== system downlink_4c2t_foldingcfr_3firs_lib/CFR_Block/PulseScaling/ScalFact ==
  v : Inport
  c : Inport  Port=2
  d : Inport  Port=3
  BitExtract : DSPBAPrim/BitExtract  primtype=bitextract  nInputs=1  nOutputs=1  omode=boolean  otype=sfix(16)  scale=1  rndmethod=Unbiased  factor=1  satmethod=Symmetric  shift_vec=[0 1 2 -1]  value=7  inPortNames=[' '; ' ';]  outPortNames=[' ']  dspbaimage=dspba_prim.jpg  text=fprintf('..%d', value);  style=Optimised  visibilities=8 + 1024  version=20090407
  Complex to Real-Iag : ComplexToRealImag
  Const2 : DSPBAPrim/Const  primtype=const  nInputs=0  nOutputs=1  omode=Inherit via internal rule  otype=sfix(16)  scale=2^-15  rndmethod=Unbiased  factor=1  satmethod=Symmetric  shift_vec=[0 1 2 -1]  value=0  inPortNames=['+'; '+';]  outPortNames=[' ']  dspbaimage=dspba_prim.jpg  text=fprintf('%s', num2str(value));  style=Optimised  visibilities=8 + 1024  floatPrecision=float32_m23  version=20120820
  Convert{,1,5..6} (4 alike) : DSPBAPrim/Convert  primtype=convert  nInputs=1  nOutputs=1  omode=Specify via dialog  otype=sfix(16)  scale=2^-15  rndmethod=Unbiased  factor=1  satmethod=None  shift_vec=[0 1 2 -1]  value=round([0:255]/17)  inPortNames=[' '; ' ';]  outPortNames=[' '; 'c']  dspbaimage=dspba_prim.jpg  text=fprintf('convert');  style=Optimised  visibilities=8+64+256+2^17  clipdetect=off  floatPrecision=float32_m23  advOptions=[]  version=20130211
  Convert10 : DSPBAPrim/Convert  primtype=convert  nInputs=1  nOutputs=1  omode=Specify via dialog  otype=ufix(8)  scale=2^-6  rndmethod=Truncate  factor=1  satmethod=None  shift_vec=[0 1 2 -1]  value=round([0:255]/17)  inPortNames=[' '; ' ';]  outPortNames=[' '; 'c']  dspbaimage=dspba_prim.jpg  text=fprintf('convert');  style=Optimised  visibilities=8+64+256+2^17  clipdetect=off  floatPrecision=float32_m23  advOptions=[]  version=20130211
  Convert8 : DSPBAPrim/Convert  primtype=convert  nInputs=1  nOutputs=1  omode=Specify via dialog  otype=ufix(16)  scale=2^-15  rndmethod=Unbiased  factor=1  satmethod=None  shift_vec=[0 1 2 -1]  value=round([0:255]/17)  inPortNames=[' '; ' ';]  outPortNames=[' '; 'c']  dspbaimage=dspba_prim.jpg  text=fprintf('convert');  style=Optimised  visibilities=8+64+256+2^17  clipdetect=off  floatPrecision=float32_m23  advOptions=[]  version=20130211
  Divide : DSPBAPrim/Divide  primtype=divide  nInputs=2  nOutputs=1  omode=Inherit via internal rule  otype=ufix(16)  scale=2^-15  rndmethod=Unbiased  factor=1  satmethod=Symmetric  shift_vec=[0 1 2 -1]  value=round([0:255]/17)  inPortNames=[' '; ' ';]  outPortNames=[' ']  dspbaimage=dspba_prim.jpg  text=fprintf('a\n----\nb');  style=Optimised  visibilities=8+2^17+2^18  floatRounding=correct  advOptions=[]  version=20130115
  Mult : DSPBAPrim/Mult  primtype=mult  nInputs=2  nOutputs=1  omode=Inherit via internal rule  otype=sfix(16)  scale=2^-15  rndmethod=Unbiased  factor=1  satmethod=Symmetric  shift_vec=[0 1 2 -1]  value=0  inPortNames=[' '; ' ';]  outPortNames=[' ']  dspbaimage=dspba_prim.jpg  text=fprintf('X');  style=Optimised  visibilities=8+2^18+2^19  floatPrecision=float32_m23  floatRounding=correct  advOptions=[]  version=20130115
  Mult1 : DSPBAPrim/Mult  primtype=mult  nInputs=2  nOutputs=1  omode=Inherit via internal rule  otype=sfix(16)  scale=2^-15  rndmethod=Unbiased  factor=1  satmethod=Symmetric  shift_vec=[0 1 2 -1]  value=0  inPortNames=[' '; ' ';]  outPortNames=[' ']  dspbaimage=dspba_prim.jpg  text=fprintf('X');  style=Optimised  visibilities=8+2^18+2^19  floatPrecision=float32_m23  floatRounding=correct  advOptions=[]  version=20130115
  Mux : DSPBAPrim/Mux  primtype=mux  nInputs=evalAionMaskParam(gcb,'value',1)+1  nOutputs=1  omode=Inherit via internal rule  otype=sfix(16)  scale=2^-15  rndmethod=Unbiased  factor=1  satmethod=Symmetric  shift_vec=[0 1 2 -1]  value=2  inPortNames=['s'; 'd0'; 'd1'; 'd2'; 'd3'; 'd4'; 'd5'; 'd6'; 'd7'; 'd8'; 'd9';]  outPortNames=[' ']  dspbaimage=dspba_prim.jpg  text=fprintf('%s', primtype);  style=Optimised  visibilities=1032  version=20131025
  One2 : DSPBAPrim/Const  primtype=const  nInputs=0  nOutputs=1  omode=Specify via dialog  otype=sfix(18)  scale=2^-14  rndmethod=Unbiased  factor=1  satmethod=Symmetric  shift_vec=[0 1 2 -1]  value=0  inPortNames=['+'; '+';]  outPortNames=[' ']  dspbaimage=dspba_prim.jpg  text=fprintf('%s', num2str(value));  style=Optimised  visibilities=8 + 1024  floatPrecision=float32_m23  version=20120820
  One5 : DSPBAPrim/Const  primtype=const  nInputs=0  nOutputs=1  omode=Specify via dialog  otype=uint(4)  scale=2^0  rndmethod=Unbiased  factor=1  satmethod=Symmetric  shift_vec=[0 1 2 -1]  value=2  inPortNames=['+'; '+';]  outPortNames=[' ']  dspbaimage=dspba_prim.jpg  text=fprintf('%s', num2str(value));  style=Optimised  visibilities=8 + 1024  floatPrecision=float32_m23  version=20120820
  Real-Imag to Complex : RealImagToComplex
  RegField : DSPBAModelBus/RegField  reg_name=cfr_Params.BaseAddr + REG.Threshold  reg_rwmode=Read/Write  reg_msb=7  reg_lsb=0  reg_mode=Specify via dialog  reg_type=ufix(8)  reg_scale=2^-6  reg_init=cfr_Params.ClipVal  reg_desc=Clipping value  reg_modal=off  reg_desc0=0  reg_desc1=0  reg_desc2=0  reg_desc3=0  reg_desc4=0  reg_desc5=0  reg_desc6=0  reg_desc7=0  SampleTime=1  version=20090407
  Shift : DSPBAPrim/Shift  primtype=shift  nInputs=2  nOutputs=1  omode=Specify via dialog  otype=sfix(16)  scale=2^-15  rndmethod=Unbiased  factor=1  satmethod=Symmetric  shift_vec=[0 1 2 -1]  value=0  inPortNames=['a'; 'b';]  outPortNames=[' ']  dspbaimage=dspba_prim.jpg  text=fprintf('a >> b');  style=Optimised  visibilities=8  version=20090407
  Shift1 : DSPBAPrim/Shift  primtype=shift  nInputs=2  nOutputs=1  omode=Specify via dialog  otype=sfix(16)  scale=2^-15  rndmethod=Unbiased  factor=1  satmethod=Symmetric  shift_vec=[0 1 2 -1]  value=0  inPortNames=['a'; 'b';]  outPortNames=[' ']  dspbaimage=dspba_prim.jpg  text=fprintf('a >> b');  style=Optimised  visibilities=8  version=20090407
  Sub1 : DSPBAPrim/Sub  primtype=sub  nInputs=2  nOutputs=1  omode=Inherit via internal rule  otype=sfix(16)  scale=2^-15  rndmethod=Unbiased  factor=1  satmethod=Symmetric  shift_vec=[0 1 2 -1]  value=0  inPortNames=['+'; '-';]  outPortNames=[' ']  dspbaimage=dspba_prim.jpg  text=fprintf('-');  style=Optimised  visibilities=8  floatRounding=correct  advOptions=[]  version=20130115
  Subsystem : Subsystem  AncestorBlock=CORDIC_lib/Subsystem  mask{stages=cfr_stages, angle_bits=cfr_angle_cord_bits, angle_frac_bits=cfr_angle_cord_fractional_bits, xy_bits=cfr_xy_cord_bits, xy_frac_bits=cfr_xy_cord_fractional_bits}
      mask prompts: angle_bits "Angle bits"; angle_frac_bits "Angle fractional bits"; xy_bits "XY bits"; xy_frac_bits "XY fractional bits"
      mask init:
      | sys = gcb;
      | 
      | % error trapping
      | if (angle_bits-angle_frac_bits)<3
      |     fprintf(['Warning (' sys ') not sufficient angle integer bits to represent full angle swing (-pi to pi)']);
      | end
      | 
      | if angle_bits < stages 
      |     fprintf(['Warning (' sys ') #angle bits < stages behaviour may be unexpected']);
      | end
      | 
      | if xy_bits < stages 
      |     fprintf(['Warning (' sys ') #xy bits < stages behaviour may be unexpected']);
      | end
      mask Display:
      | % calculate gain
      | gain = 1;
      | for i=0:stages
      |     gain = gain*(sqrt((1+2^(-2*i))));
      | end
      | color('w');image(imread('dspba_prim.jpg'));
      | fprintf('CORDIC\nRotate\n(pi to -pi)\ngain=%1.4f\niterations=%i',gain,stages+1);
      | port_label('input',1,'v_in');
      | port_label('input',2,'c_in');
      | port_label('input',3,'x_in');
      | port_label('input',4,'y_in');
      | port_label('input',5,'p_in');
      | port_label('output',1,'v_out');
      | port_label('output',2,'c_out');
      | port_label('output',3,'x_out');
      | port_label('output',4,'y_out');
      | port_label('output',5,'p_out');
  TermY{1..3,8} (4 alike) : Terminator
  qv : Outport
  qc : Outport  Port=2
  Out_c : Outport  Port=3
  wires:
  Complex to Real-Iag/2 -> Shift1/1, Convert6/1
  Sub1/1 -> Divide/1, BitExtract/1
  BitExtract/1 -> Mux/1
  RegField/1 -> Sub1/2
  Mult/1 -> Convert/1
  Complex to Real-Iag/1 -> Convert5/1, Shift/1
  Mult1/1 -> Convert1/1
  Convert5/1 -> Mult/1
  Convert6/1 -> Mult1/1
  Convert/1 -> Real-Imag to Complex/1
  Convert1/1 -> Real-Imag to Complex/2
  Const2/1 -> Mux/3
  Divide/1 -> Mux/2
  d/1 -> Complex to Real-Iag/1
  v/1 -> qv/1, Subsystem/1(av)
  c/1 -> qc/1, Subsystem/2(ac)
  Real-Imag to Complex/1 -> Out_c/1
  Mux/1 -> Convert8/1
  Convert8/1 -> Mult/2, Mult1/2
  Shift/1 -> Subsystem/3(xin)
  Shift1/1 -> Subsystem/4(yin)
  One2/1 -> Subsystem/5(pin)
  One5/1 -> Shift/2, Shift1/2
  Subsystem/3(xout) -> Convert10/1
  Convert10/1 -> Divide/2, Sub1/1
  Subsystem/1(qv) -> TermY8/1
  Subsystem/2(qc) -> TermY1/1
  Subsystem/4(yout) -> TermY2/1
  Subsystem/5(pout) -> TermY3/1

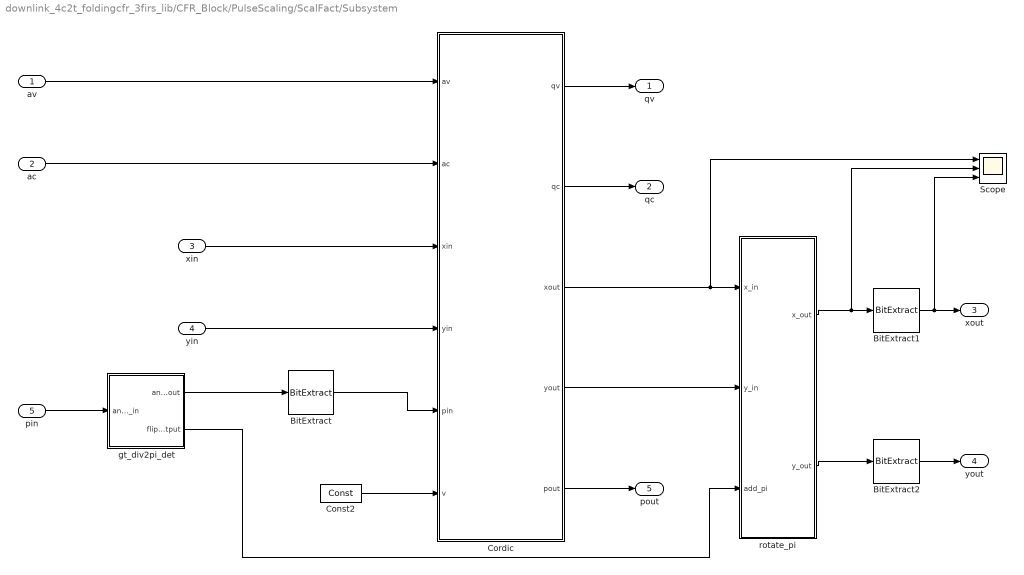
== system downlink_4c2t_foldingcfr_3firs_lib/CFR_Block/PulseScaling/ScalFact/Subsystem ==
  av : Inport
  ac : Inport  Port=2
  xin : Inport  Port=3
  yin : Inport  Port=4
  pin : Inport  Port=5
  BitExtract : DSPBAPrim/BitExtract  primtype=bitextract  nInputs=1  nOutputs=1  omode=Specify via dialog  otype=sfix(angle_bits-1)  scale=2^-angle_frac_bits  rndmethod=Unbiased  factor=1  satmethod=Symmetric  shift_vec=[0 1 2 -1]  value=0  inPortNames=[' '; ' ';]  outPortNames=[' ']  dspbaimage=dspba_prim.jpg  text=fprintf('..%d', value);  style=Optimised  visibilities=8 + 1024  version=20090407
  BitExtract1 : DSPBAPrim/BitExtract  primtype=bitextract  nInputs=1  nOutputs=1  omode=Specify via dialog  otype=sfix(xy_bits)  scale=2^-xy_frac_bits  rndmethod=Unbiased  factor=1  satmethod=Symmetric  shift_vec=[0 1 2 -1]  value=0  inPortNames=[' '; ' ';]  outPortNames=[' ']  dspbaimage=dspba_prim.jpg  text=fprintf('..%d', value);  style=Optimised  visibilities=8 + 1024  version=20090407
  BitExtract2 : DSPBAPrim/BitExtract  primtype=bitextract  nInputs=1  nOutputs=1  omode=Specify via dialog  otype=sfix(xy_bits)  scale=2^-xy_frac_bits  rndmethod=Unbiased  factor=1  satmethod=Symmetric  shift_vec=[0 1 2 -1]  value=0  inPortNames=[' '; ' ';]  outPortNames=[' ']  dspbaimage=dspba_prim.jpg  text=fprintf('..%d', value);  style=Optimised  visibilities=8 + 1024  version=20090407
  Const2 : DSPBAPrim/Const  primtype=const  nInputs=0  nOutputs=1  omode=Specify via dialog  otype=uint(1)  scale=2^0  rndmethod=Unbiased  factor=1  satmethod=Symmetric  shift_vec=[0 1 2 -1]  value=1  inPortNames=['+'; '+';]  outPortNames=[' ']  dspbaimage=dspba_prim.jpg  text=fprintf('%s', num2str(value));  style=Optimised  visibilities=8 + 1024  floatPrecision=float32_m23  version=20120820
  Cordic : Subsystem  AncestorBlock=CORDIC_lib/Cordic  mask(CORDIC range -pi/2 to pi/2){stages=stages, angle_bits=angle_bits-1, angle_frac_bits=angle_frac_bits, xy_bits=xy_bits, xy_frac_bits=xy_frac_bits}
      mask prompts: angle_bits "Angle bits"; angle_frac_bits "Angle fractional bits"; xy_bits "XY bits"; xy_frac_bits "XY fractional bits"
      mask help:
      | Primitive block implementation of CORDIC.
      | Range -pi/2 to pi/2
      |
      | See "Help" for information on parameter selection.
      mask init:
      | setup_cordic_block(stages, angle_bits, angle_frac_bits, xy_bits, xy_frac_bits);
      mask Help:
      | By default it is expected that stages = angle_bits = xy_bits also that
      | angle_frac_bits = angle_bits-2 (i.e. 2 integer angle bits)
      | 
      | It is assumed that stages <= angle_bits and stages <= xy_bits
      | 
      | Parameter description:
      | 
      | Stages (stages)
      | Number of CORDIC stages
      | Note counting starts at zero so "iterations = stages+1"
      | 
      | Angle bits (angle_bits)
      | Number of bits used to represent the angle, data format is "sfix"
      | 
      | Angle fractional bits (angle_frac_bits)
      | Number of angle bits which are fractional
      | Angle format will be "sfix[angle_bits]_[angle_frac_bits]"
      | 
      | XY bits (xy_bits)
      | Number of bits used to represent inputs x,y, data format is "sfix"
      | 
      | XY fractional bits (xy_frac_bits)
      | Number of x,y bits which are fractional
      | Format will be "sfix[xy_bits]_[xy_frac_bits]"
      | 
      | 
      | For more information on CORDIC see the following paper (from which this
      | implementation was created):
      | 
      | "A survey of CORDIC algorithms for FPGAs"
      | Ray Andraka, FPGA '98
      mask Display:
      | % calculate gain
      | gain = 1;
      | for i=0:stages
      |     gain = gain*(sqrt((1+2^(-2*i))));
      | end
      | color('w');image(imread('dspba_prim.jpg'));
      | fprintf('CORDIC\n(pi/2 to -pi/2)\ngain=%1.4f\niterations=%i',gain,stages+1);
      | 
      | port_label('input',1,'v_in');
      | port_label('input',2,'c_in');
      | port_label('input',3,'x_in');
      | port_label('input',4,'y_in');
      | port_label('input',5,'p_in');
      | port_label('input',6,'mode');
      | port_label('output',1,'v_out');
      | port_label('output',2,'c_out');
      | port_label('output',3,'x_out');
      | port_label('output',4,'y_out');
      | port_label('output',5,'p_out');
  Scope : Scope  NumInputPorts=3
  gt_div2pi_det : Subsystem  mask{angle_bits=angle_bits}
      mask prompts: angle_bits "Angle bits"
  rotate_pi : Subsystem
  qv : Outport
  qc : Outport  Port=2
  xout : Outport  Port=3
  yout : Outport  Port=4
  pout : Outport  Port=5
  wires:
  av/1 -> Cordic/1(av)
  ac/1 -> Cordic/2(ac)
  Cordic/1(qv) -> qv/1
  Cordic/2(qc) -> qc/1
  Cordic/3(xout) -> Scope/1, rotate_pi/1(x_in)
  Cordic/4(yout) -> rotate_pi/2(y_in)
  Cordic/5(pout) -> pout/1
  xin/1 -> Cordic/3(xin)
  yin/1 -> Cordic/4(yin)
  pin/1 -> gt_div2pi_det/1(angle_in)
  gt_div2pi_det/1(angle_out) -> BitExtract/1
  rotate_pi/1(x_out) -> Scope/2, BitExtract1/1
  rotate_pi/2(y_out) -> BitExtract2/1
  gt_div2pi_det/2(flip_output) -> rotate_pi/3(add_pi)
  Const2/1 -> Cordic/6(v)
  BitExtract/1 -> Cordic/5(pin)
  BitExtract1/1 -> Scope/3, xout/1
  BitExtract2/1 -> yout/1
